simulink model "pv_seul_etudiant"  (R2022a)
settings: Solver=FixedStepAuto  StartTime=0.0  StopTime=10  FixedStep=0.01  RelTol=1e-3
values from neighbouring files (symbols this model uses):
  alpharange = 0.01: 0.01 : 1    [Temperature.m]
  Irr = Irrtmp(j)    [IV.m]    (also in Temperature.m = 1000; panneauxvietnam.m = 520)
  Tpv = 273.15+25    (= 298.15)    [IV.m]    (also in Temperature.m = temptmp(j); panneauxvietnam.m)
settings Model: Creator=guillaume  LastModifiedBy=habayah
settings DebuggingCC: UnconnectedInputMsg=warning  UnconnectedOutputMsg=warning  UnconnectedLineMsg=warning
settings RTWCC: DLArmComputeVersion=19.05

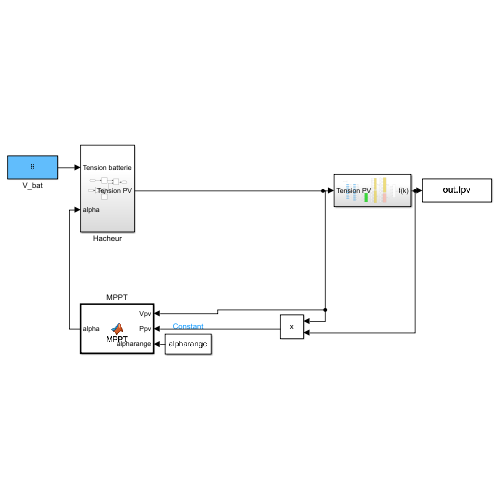
[thumbnail: Simulink's stored preview of the top-level diagram]
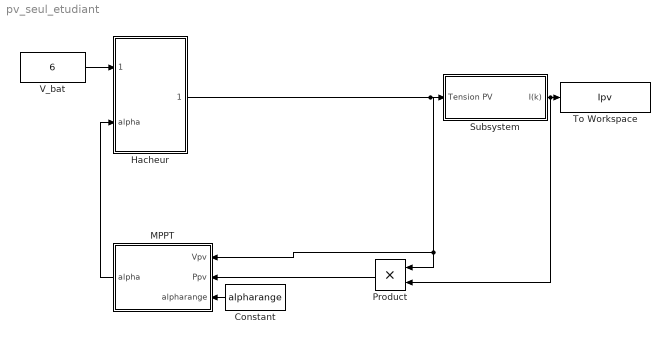
== system pv_seul_etudiant ==
  Constant : Constant  Value=alpharange
  Hacheur : Subsystem
  MPPT : MATLAB Function  TreatAsAtomicUnit=on
  Product : Product
  Subsystem : Subsystem
  To Workspace : ToWorkspace  VariableName=Ipv  SaveFormat=Timeseries  SampleTime=-1
  V_bat : Constant  Value=6
  wires:
  V_bat/1 -> Hacheur/1(Tension batterie)
  Hacheur/1(Tension PV) -> Product/1, MPPT/1(Vpv), Subsystem/1(Tension PV)
  Subsystem/1(I(k)) -> Product/2, To Workspace/1
  MPPT/1(alpha) -> Hacheur/2(alpha)
  Product/1 -> MPPT/2(Ppv)
  Constant/1 -> MPPT/3(alpharange)

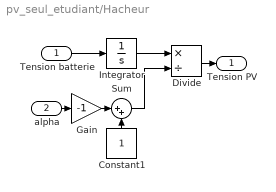
== system pv_seul_etudiant/Hacheur ==
  Tension batterie : Inport
  alpha : Inport  Port=2
  Constant1 : Constant
  Divide : Product  Inputs=*/
  Gain : Gain  Gain=-1
  Integrator : Integrator
  Sum : Sum  Inputs=|++
  Tension PV : Outport
  wires:
  alpha/1 -> Gain/1
  Divide/1 -> Tension PV/1
  Tension batterie/1 -> Integrator/1
  Integrator/1 -> Divide/1
  Gain/1 -> Sum/1
  Constant1/1 -> Sum/2
  Sum/1 -> Divide/2

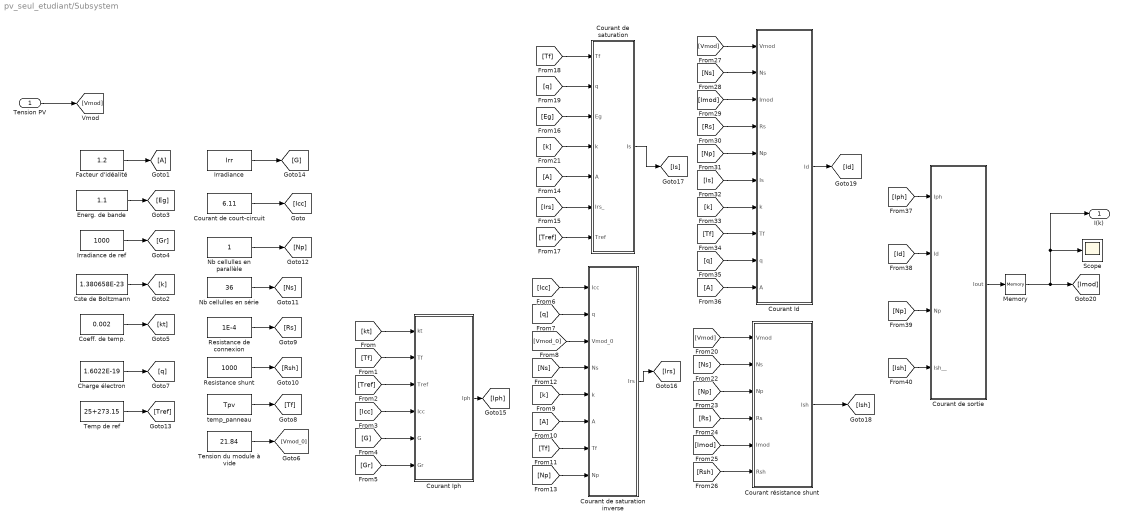
== system pv_seul_etudiant/Subsystem ==
  Tension PV : Inport
  Charge électron : Constant  Value=1.6022E-19
  Coeff. de temp. : Constant  Value=0.002
  Courant Id : Subsystem
  Courant Iph : Subsystem
  Courant de court-circuit : Constant  Value=6.11
  "Courant de saturation " : Subsystem
  Courant de saturation inverse : Subsystem
  Courant de sortie : Subsystem
  Courant résistance shunt : Subsystem
  "Cste de Boltzmann " : Constant  Value=1.380658E-23  VectorParams1D=off
  Energ. de bande : Constant  Value=1.1  VectorParams1D=off
  Facteur d'idéalité : Constant  Value=1.2
  From10 : From
  From14 : From
  From36 : From
  Goto1 : Goto
  Irradiance : Constant  Value=Irr
  Irradiance de ref : Constant  Value=1000
  Memory : Memory  InitialCondition=0.000001
  Nb cellulles en parallèle : Constant
  Nb cellulles en série : Constant  Value=36
  Resistance de connexion : Constant  Value=1E-4
  Resistance shunt : Constant  Value=1000
  Scope : Scope
  Temp de ref : Constant  Value=25+273.15
  Tension du module à vide : Constant  Value=21.84
  temp_panneau : Constant  Value=Tpv
  I(k) : Outport
  wires:
  [Icc] -> Courant Iph/4(Icc)
  [Np] -> Courant résistance shunt/3(Np)
  "Courant de saturation "/1(Is) -> [Is]
  [G] -> Courant Iph/5(G)
  Courant de saturation inverse/1(Irs) -> [Irs]
  Temp de ref/1 -> [Tref]
  Tension du module à vide/1 -> [Vmod_0]
  [k] -> "Courant de saturation "/4(k)
  [q] -> Courant de saturation inverse/2(q)
  [Tf] -> Courant Iph/2(Tf)
  From14/1 -> "Courant de saturation "/5(A)
  [Ns] -> Courant Id/2(Ns)
  Resistance shunt/1 -> [Rsh]
  [Imod] -> Courant résistance shunt/5(Imod)
  [Rs] -> Courant résistance shunt/4(Rs)
  [Vmod_0] -> Courant de saturation inverse/3("Vmod_0 ")
  [Irs] -> "Courant de saturation "/6(Irs_)
  Resistance de connexion/1 -> [Rs]
  Nb cellulles en série/1 -> [Ns]
  [Eg] -> "Courant de saturation "/3("Eg ")
  [q] -> "Courant de saturation "/2(q)
  [q] -> Courant Id/9(q)
  [Tf] -> "Courant de saturation "/1(Tf)
  From10/1 -> Courant de saturation inverse/6(A)
  [Tf] -> Courant Id/8(Tf)
  Nb cellulles en parallèle/1 -> [Np]
  [Tref] -> Courant Iph/3(Tref)
  [Tf] -> Courant de saturation inverse/7(Tf)
  Coeff. de temp./1 -> [kt]
  [Np] -> Courant de sortie/3(Np)
  [Is] -> Courant Id/6(Is)
  [k] -> Courant Id/7(k)
  Irradiance de ref/1 -> [Gr]
  [k] -> Courant de saturation inverse/5(k)
  "Cste de Boltzmann "/1 -> [k]
  [Icc] -> Courant de saturation inverse/1(Icc)
  Courant de court-circuit/1 -> [Icc]
  Tension PV/1 -> [Vmod]
  Courant Id/1(Id) -> [Id]
  [Vmod] -> Courant Id/1(Vmod)
  Courant de sortie/1(Iout) -> Memory/1
  [Ish] -> Courant de sortie/4(Ish__)
  From36/1 -> Courant Id/10(A)
  Energ. de bande/1 -> [Eg]
  [Id] -> Courant de sortie/2(Id)
  [Imod] -> Courant Id/3(Imod)
  [Vmod] -> Courant résistance shunt/1(Vmod)
  Charge électron/1 -> [q]
  [kt] -> Courant Iph/1(kt)
  Courant résistance shunt/1(Ish) -> [Ish]
  temp_panneau/1 -> [Tf]
  [Rs] -> Courant Id/4(Rs)
  [Ns] -> Courant de saturation inverse/4("Ns ")
  [Gr] -> Courant Iph/6(Gr)
  Courant Iph/1(Iph) -> [Iph]
  [Np] -> Courant de saturation inverse/8(Np)
  Facteur d'idéalité/1 -> Goto1/1
  [Iph] -> Courant de sortie/1(Iph)
  [Tref] -> "Courant de saturation "/7(Tref)
  [Rsh] -> Courant résistance shunt/6(Rsh)
  [Np] -> Courant Id/5(Np)
  [Ns] -> Courant résistance shunt/2(Ns)
  Irradiance/1 -> [G]
  Memory/1 -> Scope/1, I(k)/1, [Imod]

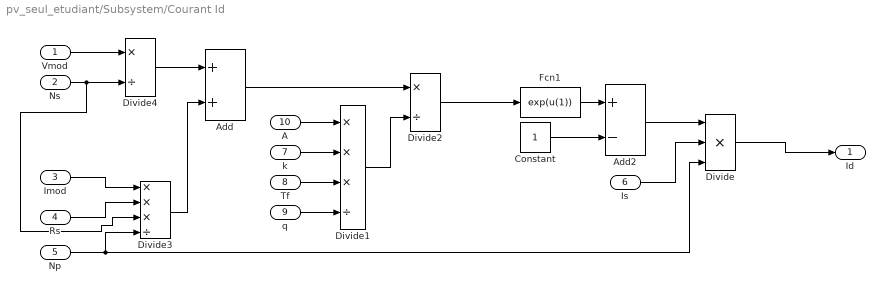
== system pv_seul_etudiant/Subsystem/Courant Id ==
  Vmod : Inport
  Ns : Inport  Port=2
  Imod : Inport  Port=3
  Rs : Inport  Port=4
  Np : Inport  Port=5
  Is : Inport  Port=6
  k : Inport  Port=7
  Tf : Inport  Port=8
  q : Inport  Port=9
  A : Inport  Port=10
  Add : Sum
  Add2 : Sum  Inputs=+-
  Constant : Constant
  Divide : Product  Inputs=***
  Divide1 : Product  Inputs=***/
  Divide2 : Product  Inputs=*/
  Divide3 : Product  Inputs=***/
  Divide4 : Product  Inputs=*/
  Fcn1 : Fcn  Expr=exp(u(1))
  Id : Outport  VectorParamsAs1DForOutWhenUnconnected=off
  wires:
  Divide/1 -> Id/1
  Vmod/1 -> Divide4/1
  Ns/1 -> Divide4/2, Divide3/3
  Divide4/1 -> Add/1
  Imod/1 -> Divide3/1
  Rs/1 -> Divide3/2
  Divide3/1 -> Add/2
  Np/1 -> Divide/3, Divide3/4
  Constant/1 -> Add2/2
  Fcn1/1 -> Add2/1
  Add2/1 -> Divide/1
  Is/1 -> Divide/2
  Divide1/1 -> Divide2/2
  Add/1 -> Divide2/1
  Divide2/1 -> Fcn1/1
  q/1 -> Divide1/4
  Tf/1 -> Divide1/3
  k/1 -> Divide1/2
  A/1 -> Divide1/1

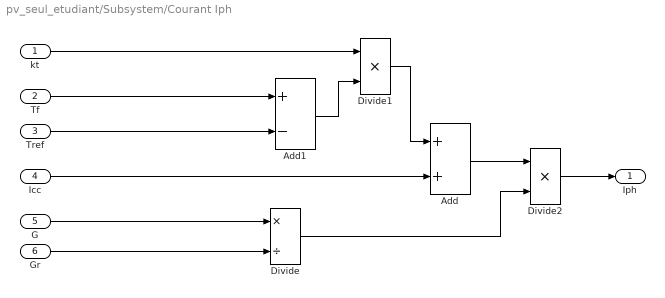
== system pv_seul_etudiant/Subsystem/Courant Iph ==
  kt : Inport
  Tf : Inport  Port=2
  Tref : Inport  Port=3
  Icc : Inport  Port=4
  G : Inport  Port=5
  Gr : Inport  Port=6
  Add : Sum
  Add1 : Sum  Inputs=+-
  Divide : Product  Inputs=*/
  Divide1 : Product  Inputs=**
  Divide2 : Product  Inputs=**
  Iph : Outport  VectorParamsAs1DForOutWhenUnconnected=off
  wires:
  Tf/1 -> Add1/1
  Tref/1 -> Add1/2
  Icc/1 -> Add/2
  G/1 -> Divide/1
  Gr/1 -> Divide/2
  Add1/1 -> Divide1/2
  kt/1 -> Divide1/1
  Divide1/1 -> Add/1
  Add/1 -> Divide2/1
  Divide2/1 -> Iph/1
  Divide/1 -> Divide2/2

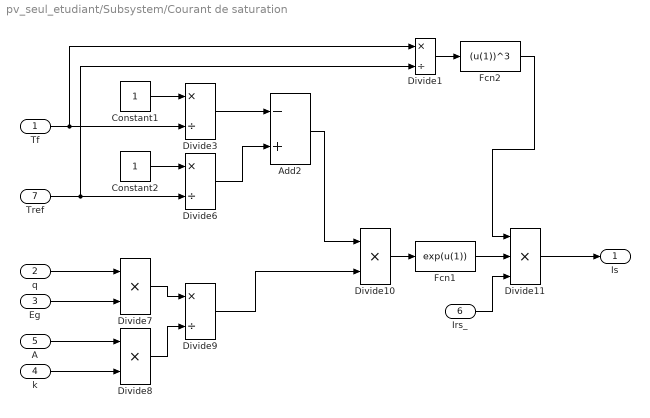
== system pv_seul_etudiant/Subsystem/Courant de saturation  ==
  Tf : Inport
  q : Inport  Port=2
  "Eg " : Inport  Port=3
  k : Inport  Port=4
  A : Inport  Port=5
  Irs_ : Inport  Port=6
  Tref : Inport  Port=7
  Add2 : Sum  Inputs=-+
  Constant1 : Constant
  Constant2 : Constant
  Divide{1,3,6,9} (4 alike) : Product  Inputs=*/
  Divide10 : Product  Inputs=**
  Divide11 : Product  Inputs=***
  Divide7 : Product  Inputs=**
  Divide8 : Product  Inputs=**
  Fcn1 : Fcn  Expr=exp(u(1))
  Fcn2 : Fcn  Expr=(u(1))^3
  Is : Outport  VectorParamsAs1DForOutWhenUnconnected=off
  wires:
  Constant1/1 -> Divide3/1
  Tf/1 -> Divide1/1, Divide3/2
  Tref/1 -> Divide1/2, Divide6/2
  Constant2/1 -> Divide6/1
  Divide3/1 -> Add2/1
  Divide6/1 -> Add2/2
  q/1 -> Divide7/1
  "Eg "/1 -> Divide7/2
  A/1 -> Divide8/1
  k/1 -> Divide8/2
  Divide7/1 -> Divide9/1
  Divide8/1 -> Divide9/2
  Add2/1 -> Divide10/1
  Divide9/1 -> Divide10/2
  Divide10/1 -> Fcn1/1
  Fcn1/1 -> Divide11/2
  Divide1/1 -> Fcn2/1
  Irs_/1 -> Divide11/3
  Fcn2/1 -> Divide11/1
  Divide11/1 -> Is/1

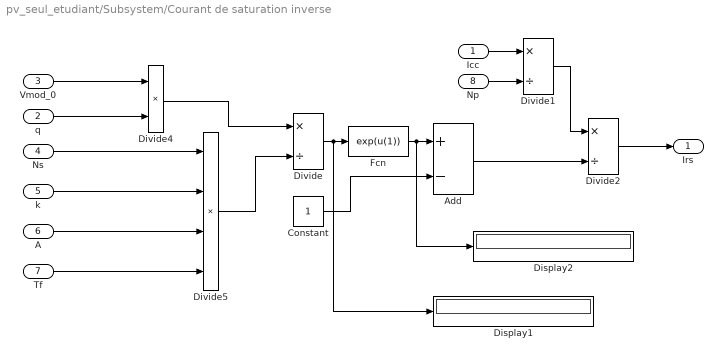
== system pv_seul_etudiant/Subsystem/Courant de saturation inverse ==
  Icc : Inport
  q : Inport  Port=2
  "Vmod_0 " : Inport  Port=3
  "Ns " : Inport  Port=4
  k : Inport  Port=5
  A : Inport  Port=6
  Tf : Inport  Port=7
  Np : Inport  Port=8
  Add : Sum  Inputs=+-
  Constant : Constant
  Display1 : Display
  Display2 : Display
  Divide : Product  Inputs=*/
  Divide1 : Product  Inputs=*/
  Divide2 : Product  Inputs=*/
  Divide4 : Product  Inputs=**
  Divide5 : Product  Inputs=****
  Fcn : Fcn  Expr=exp(u(1))
  Irs : Outport  VectorParamsAs1DForOutWhenUnconnected=off
  wires:
  Divide2/1 -> Irs/1
  "Vmod_0 "/1 -> Divide4/1
  q/1 -> Divide4/2
  "Ns "/1 -> Divide5/1
  k/1 -> Divide5/2
  A/1 -> Divide5/3
  Tf/1 -> Divide5/4
  Divide4/1 -> Divide/1
  Divide5/1 -> Divide/2
  Constant/1 -> Add/2
  Add/1 -> Divide2/2
  Icc/1 -> Divide1/1
  Np/1 -> Divide1/2
  Divide1/1 -> Divide2/1
  Divide/1 -> Display1/1, Fcn/1
  Fcn/1 -> Display2/1, Add/1

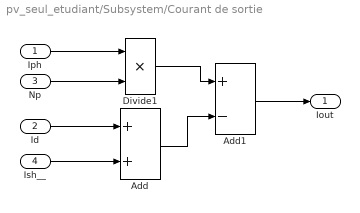
== system pv_seul_etudiant/Subsystem/Courant de sortie ==
  Iph : Inport
  Id : Inport  Port=2
  Np : Inport  Port=3
  Ish__ : Inport  Port=4
  Add : Sum
  Add1 : Sum  Inputs=+-
  Divide1 : Product  Inputs=**
  Iout : Outport  VectorParamsAs1DForOutWhenUnconnected=off
  wires:
  Iph/1 -> Divide1/1
  Np/1 -> Divide1/2
  Divide1/1 -> Add1/1
  Add1/1 -> Iout/1
  Id/1 -> Add/1
  Ish__/1 -> Add/2
  Add/1 -> Add1/2

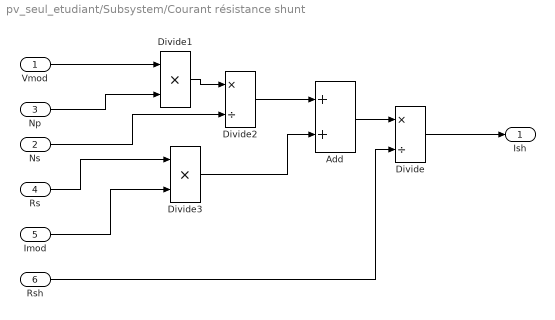
== system pv_seul_etudiant/Subsystem/Courant résistance shunt ==
  Vmod : Inport
  Ns : Inport  Port=2
  Np : Inport  Port=3
  Rs : Inport  Port=4
  Imod : Inport  Port=5
  Rsh : Inport  Port=6
  Add : Sum
  Divide : Product  Inputs=*/
  Divide1 : Product  Inputs=**
  Divide2 : Product  Inputs=*/
  Divide3 : Product  Inputs=**
  Ish : Outport  VectorParamsAs1DForOutWhenUnconnected=off
  wires:
  Divide/1 -> Ish/1
  Vmod/1 -> Divide1/1
  Np/1 -> Divide1/2
  Divide1/1 -> Divide2/1
  Ns/1 -> Divide2/2
  Divide2/1 -> Add/1
  Imod/1 -> Divide3/2
  Rs/1 -> Divide3/1
  Divide3/1 -> Add/2
  Add/1 -> Divide/1
  Rsh/1 -> Divide/2

== matlab function pv_seul_etudiant/MPPT ==
  data: Vpv input; alpha output; Ppv input; alpharange input
function alpha = MPPT(Vpv,Ppv,alpharange)


Pnew=Ppv;
persistent i;
persistent Pold;

if Pnew-Pold>0
    if Vnew-Vold>0
        i=i+1;
    else
        i=i-1;
    end

else
    if Vnew-Vold>0
        i=i-1;
    else
        i=i+1;
    end
end

    
if i>length(alpharange)
    i=length(alpharange);
elseif i<1
    i=1;
end

Pold= Pnew;

alpha=alpharange(i)
